simulink model "pid12"  (R2018a)
settings: Solver=VariableStepAuto  StartTime=0.0  StopTime=200  FixedStep=50e-3  RelTol=1e-3
libraries: simulink x1
settings Model: Creator=Dani  LastModifiedBy=Dani

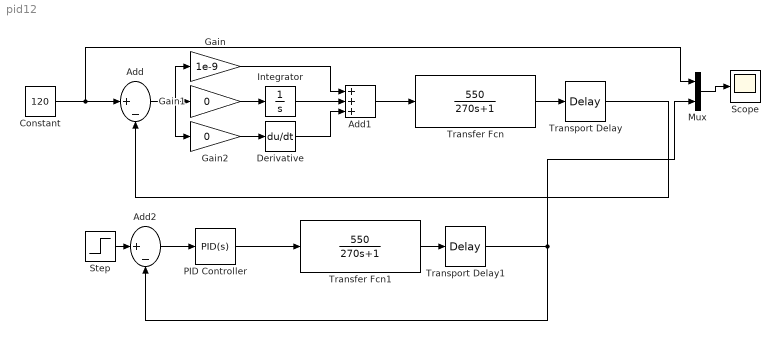
== system pid12 ==
  Add : Sum  Inputs=|+-
  Add1 : Sum  Inputs=3
  Add2 : Sum  Inputs=|+-
  Constant : Constant  Value=120
  Derivative : Derivative  CoefficientInTFapproximation=1
  Gain : Gain  Gain=1e-9
  Gain1 : Gain  Gain=0
  Gain2 : Gain  Gain=0
  Integrator : Integrator
  Mux : Mux  Inputs=2
  PID Controller : simulink/Continuous/PID Controller  Controller=PID  TimeDomain=Continuous-time  SampleTime=-1  IntegratorMethod=Forward Euler  FilterMethod=Forward Euler  Form=Ideal  UseFilter=on  ControllerParametersSource=internal  P=3.7  I=0.0041  D=7.5  N=100  InitialConditionSource=internal  InitialConditionForIntegrator=0  InitialConditionForFilter=0  ExternalReset=none  LimitOutput=off  UpperSaturationLimit=inf  LowerSaturationLimit=-inf  LinearizeAsGain=on  AntiWindupMode=none  Kb=1  TrackingMode=off  Kt=1  PParamMin=[]  PParamMax=[]  IParamMin=[]  IParamMax=[]  DParamMin=[]  DParamMax=[]  NParamMin=[]  NParamMax=[]  KbParamMin=[]  KbParamMax=[]  KtParamMin=[]  KtParamMax=[]  POutMin=[]  POutMax=[]  IOutMin=[]  IOutMax=[]  DOutMin=[]  DOutMax=[]  NOutMin=[]  NOutMax=[]  KbOutMin=[]  KbOutMax=[]  KtOutMin=[]  KtOutMax=[]  IntegratorOutMin=[]  IntegratorOutMax=[]  FilterOutMin=[]  FilterOutMax=[]  SumOutMin=[]  SumOutMax=[]  SumI1OutMin=[]  SumI1OutMax=[]  SumI2OutMin=[]  SumI2OutMax=[]  SumI3OutMin=[]  SumI3OutMax=[]  SumDOutMin=[]  SumDOutMax=[]  SaturationOutMin=[]  SaturationOutMax=[]  IntegratorContinuousStateAttributes=''  IntegratorStateMustResolveToSignalObject=off  IntegratorRTWStateStorageClass=Auto  FilterContinuousStateAttributes=''  FilterStateMustResolveToSignalObject=off  FilterRTWStateStorageClass=Auto  DifferentiatorICPrevScaledInput=0  DifferentiatorOutMin=[]  DifferentiatorOutMax=[]  FilterDiffOutCoefMin=[]  FilterDiffOutCoefMax=[]  SumDenOutMin=[]  SumDenOutMax=[]  SumNumOutMin=[]  SumNumOutMax=[]  ReciprocalOutMin=[]  ReciprocalOutMax=[]  DivideOutMin=[]  DivideOutMax=[]  TunerSelectOption=Transfer Function Based (PID Tuner App)
  Scope : Scope
  Step : Step  SampleTime=0
  Transfer Fcn : TransferFcn  Numerator=[550]  Denominator=[270 1]
  Transfer Fcn1 : TransferFcn  Numerator=[550]  Denominator=[270 1]
  Transport Delay : TransportDelay  DelayTime=40
  Transport Delay1 : TransportDelay  DelayTime=30
  wires:
  Constant/1 -> Add/1, Mux/1
  Transfer Fcn/1 -> Transport Delay/1
  Transport Delay/1 -> Add/2
  Mux/1 -> Scope/1
  Integrator/1 -> Add1/2
  Derivative/1 -> Add1/3
  Add/1 -> Gain2/1, Gain1/1, Gain/1
  Gain/1 -> Add1/1
  Gain1/1 -> Integrator/1
  Gain2/1 -> Derivative/1
  Add1/1 -> Transfer Fcn/1
  PID Controller/1 -> Transfer Fcn1/1
  Step/1 -> Add2/1
  Add2/1 -> PID Controller/1
  Transfer Fcn1/1 -> Transport Delay1/1
  Transport Delay1/1 -> Mux/2, Add2/2
